simulink model "modeloSimulink"  (R2018b)
settings: Solver=ode4  StartTime=0.0  StopTime=100  FixedStep=0.04  RelTol=1e-3
libraries: simulink x9, Controllers x1
settings Model: Creator=root  LastModifiedBy=root

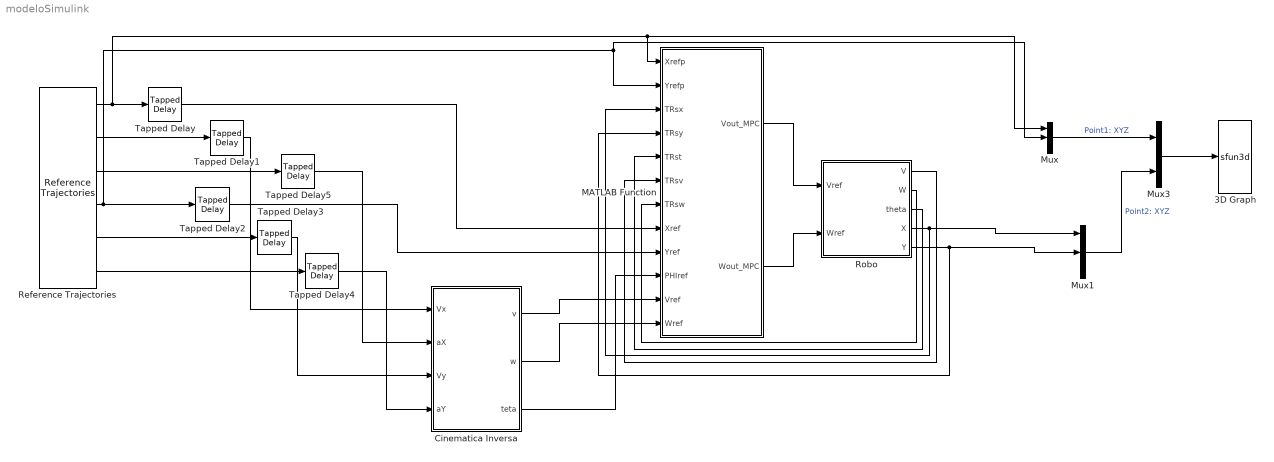
== system modeloSimulink ==
  3D Graph : S-Function  LoadFcn=if exist('sfun3d','file'), sfun3d([],[],[],'LoadBlock'); end  FunctionName=sfun3d  Parameters=ax,T,np,cp,gd,ls,mk,mx,hd,tb  SFunctionDeploymentMode=off  EnableBusSupport=off  mask(3D Graph){np=2, ax=[-4 4 -4 4 -3 3], mx=1e4, T=0.04, cp=[0 0 1], gd=on, hd=off, tb=on, ls=-, mk=none}
      mask prompts: np "Number of moving points (lines)"; ax "Range: [xmin xmax  ymin ymax zmin zmax]"; mx "Max number of points in each line"; T "Sampling Time"; cp "Camera position (use [0 0 1] for 2D XY view)"; gd "Grid (on|off)"; hd "HeadMarkers (on|off)"; tb "Toolbar (on|off)"; ls "LineStyle"; mk "LineMarker"
      mask help:
      | This block plots the position of several points in the XYZ space. The input contains the coordinates of all the points (x1,y1,z1,x2,y2,z2,...).
      | The number of moving points (lines), the XYZ ranges, sampling time, camera position, and grid (among other things) can be set as mask parameters.
      settings: CopyFcn=if exist('sfun3d','file'), sfun3d([],[],[],'CopyBlock'); end  DeleteFcn=if exist('sfun3d','file'), sfun3d([],[],[],'DeleteBlock'); end  NameChangeFcn=if exist('sfun3d','file'), sfun3d([],[],[],'NameChange'); end
      mask Help:
      | This block plots the position of several points in the XYZ space. The input contains the coordinates of all the points (x1,y1,z1,x2,y2,z2,...).
      | The number of moving points (lines), the XYZ ranges, sampling time, camera position, and grid (among other things) can be set as mask parameters.
      mask TypeOptions ls: - | -- | : | -. | none
      mask TypeOptions mk: none | . | + | o | * | x | square | diamond | v | ^ | > | < | pentagram | hexagram
      mask Display: plot([.05 .95 .95 .05 .05],[.45 .45 .95 .95 .45], 0.5+cos(0:0.1:2*pi)*0.3,0.7+sin(0:0.1:2*pi)*0.2)
  "Cinematica Inversa " : MATLAB Function  TreatAsAtomicUnit=on
  MATLAB Function : MATLAB Function  TreatAsAtomicUnit=on
  Mux : Mux  Inputs=3
  Mux1 : Mux  Inputs=3
  Mux3 : Mux  Inputs=2
  Reference Trajectories : Controllers/Reference Trajectories  trajectory_type=2  wf=0.10  raio_ref_1=1  delta_raio=0  t_delta_raio=60  xd=[1, -1.5]
  Robo : Subsystem
  Tapped Delay{,1..5} (6 alike) : simulink/Discrete/Tapped Delay  vinit=0.0  samptime=-1  NumDelays=1  DelayOrder=Oldest  includeCurrent=off
  wires:
  Robo/1(V) -> MATLAB Function/6(TRsv)
  Robo/2(W) -> MATLAB Function/7(TRsw)
  Robo/4(X) -> MATLAB Function/3(TRsx), Mux1/1
  Robo/5(Y) -> MATLAB Function/4(TRsy), Mux1/2
  MATLAB Function/2(Wout_MPC) -> Robo/2("Wref ")
  MATLAB Function/1(Vout_MPC) -> Robo/1("Vref ")
  Mux3/1 -> 3D Graph/1
  Mux1/1 -> Mux3/2  "Point2: XYZ"
  Mux/1 -> Mux3/1  "Point1: XYZ"
  Reference Trajectories/1 -> Tapped Delay/1, MATLAB Function/1(Xrefp), Mux/1
  Reference Trajectories/4 -> Tapped Delay2/1, MATLAB Function/2(Yrefp), Mux/2
  Robo/3(theta) -> MATLAB Function/5(TRst)
  Reference Trajectories/2 -> Tapped Delay1/1
  Reference Trajectories/5 -> Tapped Delay3/1
  Reference Trajectories/6 -> Tapped Delay4/1
  Reference Trajectories/3 -> Tapped Delay5/1
  Tapped Delay/1 -> MATLAB Function/8(Xref)
  Tapped Delay2/1 -> MATLAB Function/9(Yref)
  "Cinematica Inversa "/1(v) -> MATLAB Function/11(Vref)
  "Cinematica Inversa "/3(teta) -> MATLAB Function/10(PHIref)
  "Cinematica Inversa "/2(w) -> MATLAB Function/12(Wref)
  Tapped Delay4/1 -> "Cinematica Inversa "/4(aY)
  Tapped Delay3/1 -> "Cinematica Inversa "/3(Vy)
  Tapped Delay5/1 -> "Cinematica Inversa "/2(aX)
  Tapped Delay1/1 -> "Cinematica Inversa "/1(Vx)

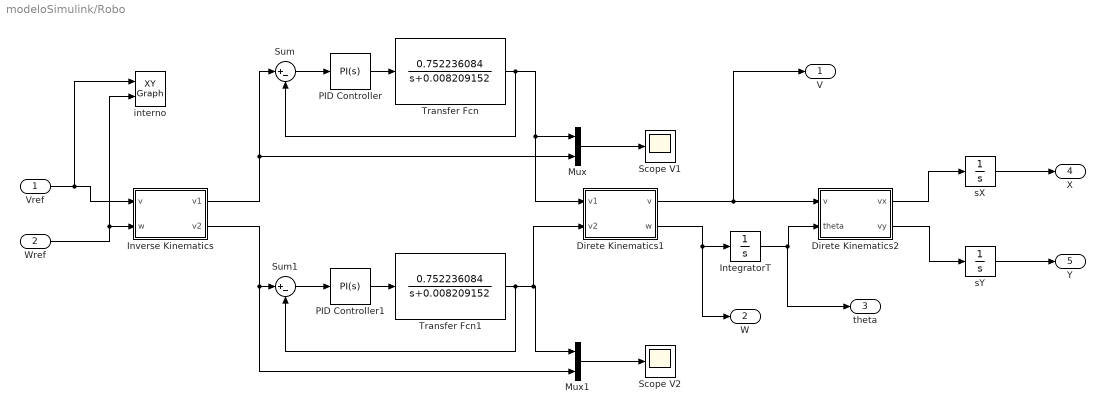
== system modeloSimulink/Robo ==
  "Vref " : Inport
  "Wref " : Inport  Port=2
  Direte Kinematics1 : MATLAB Function  TreatAsAtomicUnit=on
  Direte Kinematics2 : MATLAB Function  TreatAsAtomicUnit=on
  IntegratorT : Integrator
  Inverse Kinematics : MATLAB Function  TreatAsAtomicUnit=on
  Mux : Mux  Inputs=2
  Mux1 : Mux  Inputs=2
  PID Controller : simulink/Continuous/PID Controller  Controller=PI  Form=Parallel  TimeDomain=Continuous-time  SampleTime=-1  IntegratorMethod=Forward Euler  FilterMethod=Forward Euler  ControllerParametersSource=internal  P=13.68  I=0.87  D=0  UseFilter=on  N=100  TunerSelectOption=Transfer Function Based (PID Tuner App)  InitialConditionSource=internal  InitialConditionForIntegrator=0  InitialConditionForFilter=0  DifferentiatorICPrevScaledInput=0  ExternalReset=none  TrackingMode=off  Kt=1  LimitOutput=off  UpperSaturationLimit=inf  LowerSaturationLimit=-inf  LinearizeAsGain=on  AntiWindupMode=none  Kb=1  POutMin=[]  POutMax=[]  IOutMin=[]  IOutMax=[]  DOutMin=[]  DOutMax=[]  NOutMin=[]  NOutMax=[]  SumOutMin=[]  SumOutMax=[]  SaturationOutMin=[]  SaturationOutMax=[]  PParamMin=[]  PParamMax=[]  IParamMin=[]  IParamMax=[]  DParamMin=[]  DParamMax=[]  NParamMin=[]  NParamMax=[]  KbParamMin=[]  KbParamMax=[]  KtParamMin=[]  KtParamMax=[]  KbOutMin=[]  KbOutMax=[]  KtOutMin=[]  KtOutMax=[]  IntegratorOutMin=[]  IntegratorOutMax=[]  FilterOutMin=[]  FilterOutMax=[]  SumI1OutMin=[]  SumI1OutMax=[]  SumI2OutMin=[]  SumI2OutMax=[]  SumI3OutMin=[]  SumI3OutMax=[]  SumI4OutMin=[]  SumI4OutMax=[]  SumDOutMin=[]  SumDOutMax=[]  DifferentiatorOutMin=[]  DifferentiatorOutMax=[]  FilterDiffOutCoefMin=[]  FilterDiffOutCoefMax=[]  ReciprocalOutMin=[]  ReciprocalOutMax=[]  SumDenOutMin=[]  SumDenOutMax=[]  SumNumOutMin=[]  SumNumOutMax=[]  DivideOutMin=[]  DivideOutMax=[]  IntegratorContinuousStateAttributes=''  IntegratorStateMustResolveToSignalObject=off  IntegratorRTWStateStorageClass=Auto  FilterContinuousStateAttributes=''  FilterStateMustResolveToSignalObject=off  FilterRTWStateStorageClass=Auto  ParallelPVariant=InternalParameters  IdealPVariant=Disabled  IVariant=InternalParameters  DVariant=Disabled  IntegratorVariant=Continuous  SatVariant=Disabled  AWVariant=Passthrough  PCopyVariant=Disabled  TRVariant=Disabled  FdbkBlocksVariant=Forward  IdealPFdbkVariant=Disabled  SatFdbkVariant=Disabled  DerivativeFilterVariant=Disabled  NVariant=Disabled  NCopyVariant=Disabled_SignalSpec  FilterICVariant=Disabled  IntegratorICVariant=InternalICs  ExternalResetVariant=Disabled  TRSumVariant=Passthrough  SumFdbkVariant=Disabled  SumVariant=Sum_PI
  PID Controller1 : simulink/Continuous/PID Controller  Controller=PI  Form=Parallel  TimeDomain=Continuous-time  SampleTime=-1  IntegratorMethod=Forward Euler  FilterMethod=Forward Euler  ControllerParametersSource=internal  P=13.68  I=0.87  D=0  UseFilter=on  N=100  TunerSelectOption=Transfer Function Based (PID Tuner App)  InitialConditionSource=internal  InitialConditionForIntegrator=0  InitialConditionForFilter=0  DifferentiatorICPrevScaledInput=0  ExternalReset=none  TrackingMode=off  Kt=1  LimitOutput=off  UpperSaturationLimit=inf  LowerSaturationLimit=-inf  LinearizeAsGain=on  AntiWindupMode=none  Kb=1  POutMin=[]  POutMax=[]  IOutMin=[]  IOutMax=[]  DOutMin=[]  DOutMax=[]  NOutMin=[]  NOutMax=[]  SumOutMin=[]  SumOutMax=[]  SaturationOutMin=[]  SaturationOutMax=[]  PParamMin=[]  PParamMax=[]  IParamMin=[]  IParamMax=[]  DParamMin=[]  DParamMax=[]  NParamMin=[]  NParamMax=[]  KbParamMin=[]  KbParamMax=[]  KtParamMin=[]  KtParamMax=[]  KbOutMin=[]  KbOutMax=[]  KtOutMin=[]  KtOutMax=[]  IntegratorOutMin=[]  IntegratorOutMax=[]  FilterOutMin=[]  FilterOutMax=[]  SumI1OutMin=[]  SumI1OutMax=[]  SumI2OutMin=[]  SumI2OutMax=[]  SumI3OutMin=[]  SumI3OutMax=[]  SumI4OutMin=[]  SumI4OutMax=[]  SumDOutMin=[]  SumDOutMax=[]  DifferentiatorOutMin=[]  DifferentiatorOutMax=[]  FilterDiffOutCoefMin=[]  FilterDiffOutCoefMax=[]  ReciprocalOutMin=[]  ReciprocalOutMax=[]  SumDenOutMin=[]  SumDenOutMax=[]  SumNumOutMin=[]  SumNumOutMax=[]  DivideOutMin=[]  DivideOutMax=[]  IntegratorContinuousStateAttributes=''  IntegratorStateMustResolveToSignalObject=off  IntegratorRTWStateStorageClass=Auto  FilterContinuousStateAttributes=''  FilterStateMustResolveToSignalObject=off  FilterRTWStateStorageClass=Auto  ParallelPVariant=InternalParameters  IdealPVariant=Disabled  IVariant=InternalParameters  DVariant=Disabled  IntegratorVariant=Continuous  SatVariant=Disabled  AWVariant=Passthrough  PCopyVariant=Disabled  TRVariant=Disabled  FdbkBlocksVariant=Forward  IdealPFdbkVariant=Disabled  SatFdbkVariant=Disabled  DerivativeFilterVariant=Disabled  NVariant=Disabled  NCopyVariant=Disabled_SignalSpec  FilterICVariant=Disabled  IntegratorICVariant=InternalICs  ExternalResetVariant=Disabled  TRSumVariant=Passthrough  SumFdbkVariant=Disabled  SumVariant=Sum_PI
  Scope V1 : Scope
  Scope V2 : Scope
  Sum : Sum  Inputs=|+-
  Sum1 : Sum  Inputs=|+-
  Transfer Fcn : TransferFcn  Numerator=[0.752236084]  Denominator=[1 0.008209152]
  Transfer Fcn1 : TransferFcn  Numerator=[0.752236084]  Denominator=[1 0.008209152]
  interno : simulink/Sinks/XY Graph  xmin=-1  xmax=1  ymin=-1  ymax=1  st=-1
  sX : Integrator
  sY : Integrator
  V : Outport
  W : Outport  Port=2
  theta : Outport  Port=3
  X : Outport  Port=4
  Y : Outport  Port=5
  wires:
  Sum/1 -> PID Controller/1
  PID Controller/1 -> Transfer Fcn/1
  Transfer Fcn/1 -> Direte Kinematics1/1(v1), Mux/1, Sum/2
  Inverse Kinematics/1(v1) -> Sum/1, Mux/2
  Mux/1 -> Scope V1/1
  Mux1/1 -> Scope V2/1
  PID Controller1/1 -> Transfer Fcn1/1
  Sum1/1 -> PID Controller1/1
  Transfer Fcn1/1 -> Direte Kinematics1/2(v2), Mux1/1, Sum1/2
  Inverse Kinematics/2(v2) -> Mux1/2, Sum1/1
  Direte Kinematics1/1(v) -> Direte Kinematics2/1(v), V/1
  Direte Kinematics1/2(w) -> W/1, IntegratorT/1
  IntegratorT/1 -> theta/1, Direte Kinematics2/2(theta)
  Direte Kinematics2/2(vy) -> sY/1
  Direte Kinematics2/1(vx) -> sX/1
  sX/1 -> X/1
  sY/1 -> Y/1
  "Vref "/1 -> interno/1, Inverse Kinematics/1(v)
  "Wref "/1 -> interno/2, Inverse Kinematics/2(w)

== matlab function modeloSimulink/Robo/Direte Kinematics1 ==
  data: v1 input; v output; v2 input; w output
%function y = fcn(u)
function [v,w] = fcn(v1,v2)
    L = 2 * 0.17;
    v = (v1 + v2)/2;
    w = (v1 - v2)/L;
end

== matlab function modeloSimulink/Robo/Inverse Kinematics ==
  data: v input; v1 output; w input; v2 output
%function y = fcn(u)
function [v1,v2] = fcn(v,w)
    L = 2 * 0.17;
    v1 = v - w * L/2;
    v2 = v + w * L/2;
end

== matlab function modeloSimulink/Robo/Direte Kinematics2 ==
  data: v input; vx output; theta input; vy output
%function y = fcn(u)
function [vx,vy] = fcn(v,theta)
    vx = v * cos(deg2rad(theta));
    vy = v * sin(deg2rad(theta));
end

== matlab function modeloSimulink/MATLAB Function ==
  data: Xrefp input; Vout_MPC output; Yrefp input; TRsx input; TRsy input; TRst input; TRsv input; TRsw input; Xref input; Yref input; PHIref input; Vref input; Wref input; Wout_MPC output
function [Vout_MPC,Wout_MPC]=MPC(Xrefp,Yrefp,TRsx,TRsy,TRst,TRsv,TRsw,Xref,Yref,PHIref,Vref,Wref)
    
    



end

== matlab function modeloSimulink/Cinematica Inversa  ==
  data: Vx input; v output; aX input; Vy input; aY input; w output; teta output
function [v,w,teta] = fnc(Vx, aX, Vy, aY)
    

end;
